simulink model "BTB_Case_v1"  (R2021a)
settings: Solver=FixedStepDiscrete  StartTime=0.0  StopTime=24  FixedStep=Ts_Power  RelTol=1e-3
InitFcn:
  | %Simulation parameters
  | Ts_Power = 50e-6;
  | Ts_Control = 50e-6;
  | Ts_sec = 0.05;
  | 
  | %MV Grid parameters
  | U1n = 20e3;
  | f = 50;
  | omega = 2*pi*50;
  | 
  | 
  | %LCL filter parameters
  | L_t = 100e-6;
  | C = 173e-6;
  | L_s = 100e-6;
  | R_d = 0.086;
  | R_t = omega*L_t/100;
  | R_s = omega*L_s/100;
  | 
  | %Capacitance of the DC bus
  | Cdc = 5.88e-3;
  | Rdc = 0.00001;
  | 
  | %Coupling transformers parameters
  | U2n = 400;
  | Sn1 = 3e6;
  | 
  | %Primary Subestation parameters
  | Un = 110e3;
  | Sn = 30e6;
  | 
  | %Feeder parameters
  | Le_line_1 = 12; %length km
  | R_line_1 = (0.337)*Le_line_1; %Resistance ohms
  | X_line_1 = (0.358)*Le_line_1; %Reactance ohms
  | L_line_1 = X_line_1/omega;%Inductance H
  | 
  | Le_line_2 = 10; %length km
  | R_line_2 = (0.337)*Le_line_2; %Resistance ohms
  | X_line_2 = (0.358)*Le_line_2; %Reactance ohms
  | L_line_2 = X_line_2/omega; %Inductance H
  | 
  | %PLL parameters
  | K_p_pll = 1.8;
  | K_i_pll = 1.8/0.00251;
  | 
  | %Current control loop gains
  | tau_c = 3e-3;
  | L = L_t + L_s;
  | R =R_t + R_s;
  | Kp = L/tau_c;
  | Ki = R/tau_c;
  | 
  | %DC bus voltage control loop gains
  | tau_dc = 3*tau_c;
  | 
  | %Q-V primary control loop
  | RQ = 0.15; %Q-V regulation constant
  | 
  | %24-hours household profile pu
  | t_profile = [0:1:24].';
  | p_profile_h = [0.26 0.2 0.19 0.19 0.19 0.25 0.4 0.6 0.64 0.64 0.67 0.6 0.73 0.63 0.57 0.5 0.47 0.65 0.8 0.93 0.82 0.67 0.55 0.38 0.26].';
  | fdp_h = 0.87;
  | fi_h = acos(fdp_h);
  | q_profile_h = p_profile_h*tan(fi_h);
  | S_h = 3e6;
  | 
  | %24-hours industrial profile pu
  | p_profile_i = [0.33 0.32 0.29 0.32 0.37 0.45 0.67 0.88 1 0.99 1 0.79 0.83 0.83 0.83 0.8 0.55 0.65 0.5 0.46 0.41 0.4 0.36 0.36 0.33].';
  | fdp_i = 0.98;
  | fi_i = acos(fdp_h);
  | q_profile_i = p_profile_i*tan(fi_i);
  | S_i = 3e6;
  | 
  | %24-hours PV profile pu
  | p_profile_pv = [0 0 0 0 0 0 0 0 0 0.03 0.12 0.14 0.15 0.12 0.11 0.10 0.09 0.07 0.04 0 0 0 0 0 0].'*1/0.15;
  | S_pv = 6e6;
  | 
  | %24-hours WT profile pu
  | p_profile_wt = [0.9 0.9 1.1 1 0.9 1.1 1.25 1 0.9 0.8 0.9 0.9 1 0.8 1.5 1.3 1.2 1.2 1 0.7 1.2 0.9 1.3 1.4 0.9].'*1/1.5;
  | S_wt= 8e6;
undefined symbols (not defined in the file): D11, Delta, DiscIntNeverNeededParam, V
libraries: spsThreePhaseSeriesRLCBranchLib x16, spsThreePhaseVIMeasurementLib x13, spsRMSLib x10, simulink x6, spsSeriesRLCBranchLib x4, spsThreePhaseTransformerTwoWindingsLib x4, spsThreePhaseDynamicLoadLib x4, spsPower3phInstantaneousLib x3, eeGeneralControl x2, spsUniversalBridgeLib x2, spsVoltageMeasurementLib x2, spsThreePhaseSourceLib x1
(part 1 of 2)
settings Model: Creator=Manuel  LastModifiedBy=Manuel_Barragan

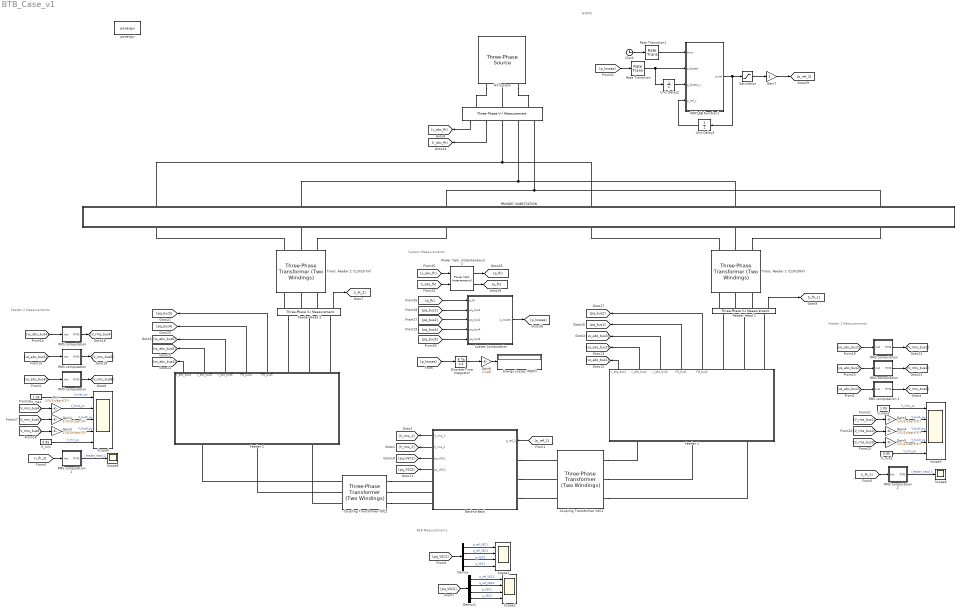
== system BTB_Case_v1 ==
  note: Feeder 2 Measurements
  note: Feeder 1 Measurements
  note: System Measurements
  note: A-DMS
  note: B2B Measurements
  " " : spsThreePhaseVIMeasurementLib/Three-Phase V-I Measurement  VoltageMeasurement=phase-to-ground  SetLabelV=off  LabelV=Vabc  Vpu=off  VpuLL=off  CurrentMeasurement=yes  SetLabelI=off  LabelI=Iabc  Ipu=off  Pbase=100e6  Vbase=500e3  OutputType=Complex  PhasorSimulation=off  PSBequivalent=0
  Back-to-Back : Subsystem
  Clock : Clock
  "Coupling Transformer VSC1 " : spsThreePhaseTransformerTwoWindingsLib/Three-Phase Transformer (Two Windings)  Winding1Connection=Delta (D11)  Winding2Connection=Yg  CoreType=Three single-phase transformers  SetSaturation=off  Hysteresis=off  DataFile='hysteresis'  SetInitialFlux=off  Measurements=None  UNITS=pu  NominalPower=[ Sn1 , f ]  Winding1=[ U1n , 0.002 , 0.08 ]  Winding2=[ U2n , 0.002 , 0.08 ]  Rm=500  Lm=500  L0=0.5  Saturation=[ 0,0 ; 0.0024,1.2 ; 1.0,1.52 ]  InitialFluxes=[ 0.8 , -0.8 , 0.7 ]  BreakLoop=off  DiscreteSolver=Trapezoidal iterative  DataType=off  TransfoNumber=1
  Coupling Transformer VSC2 : spsThreePhaseTransformerTwoWindingsLib/Three-Phase Transformer (Two Windings)  Winding1Connection=Delta (D11)  Winding2Connection=Yg  CoreType=Three single-phase transformers  SetSaturation=off  Hysteresis=off  DataFile='hysteresis'  SetInitialFlux=off  Measurements=None  UNITS=pu  NominalPower=[ Sn1 , f ]  Winding1=[ U1n , 0.002 , 0.08 ]  Winding2=[ U2n , 0.002 , 0.08 ]  Rm=500  Lm=500  L0=0.5  Saturation=[ 0,0 ; 0.0024,1.2 ; 1.0,1.52 ]  InitialFluxes=[ 0.8 , -0.8 , 0.7 ]  BreakLoop=off  DiscreteSolver=Trapezoidal iterative  DataType=off  TransfoNumber=1
  Demux : Demux
  Demux1 : Demux
  Discrete-Time Integrator : DiscreteIntegrator  SampleTime=Ts_Control  ICPrevOutput=DiscIntNeverNeededParam  ICPrevScaledInput=DiscIntNeverNeededParam
  Energy Losses (MWh) : Display
  Feeder 1 : Subsystem
  Feeder 2 : Subsystem
  Feeder Head 1 : spsThreePhaseVIMeasurementLib/Three-Phase V-I Measurement  VoltageMeasurement=no  SetLabelV=off  LabelV=Vabc  Vpu=off  VpuLL=off  CurrentMeasurement=yes  SetLabelI=off  LabelI=Iabc  Ipu=off  Pbase=100e6  Vbase=500e3  OutputType=Complex  PhasorSimulation=off  PSBequivalent=0
  Feeder Head 2 : spsThreePhaseVIMeasurementLib/Three-Phase V-I Measurement  VoltageMeasurement=no  SetLabelV=off  LabelV=Vabc  Vpu=off  VpuLL=off  CurrentMeasurement=yes  SetLabelI=off  LabelI=Iabc  Ipu=off  Pbase=100e6  Vbase=500e3  OutputType=Complex  PhasorSimulation=off  PSBequivalent=0
  Gain{,1..5} (6 alike) : Gain  Gain=1/(U1n/sqrt(3))
  Gain6 : Gain  Gain=1/1e6
  Gain7 : Gain
  HV System : spsThreePhaseSourceLib/Three-Phase Source  InternalConnection=Yg  VoltagePhases=off  Voltage=Un  PhaseAngle=0  Voltage_phases=[25e3 25e3 25e3]/sqrt(3)  PhaseAngles_phases=[0 -120 +120]  Frequency=f  NonIdealSource=off  SpecifyImpedance=on  Resistance=0.8929  Inductance=16.58e-3  ShortCircuitLevel=100e6  BaseVoltage=V  XRratio=7  BusType=swing  Pref=10e3  Qref=0  Prefabc=[10e3, 10e3, 10e3]  Qrefabc=[0, 0, 0]  Qmin=-inf  Qmax=inf
  Losses Computation : MATLAB Function  TreatAsAtomicUnit=on
  MATLAB Function1 : MATLAB Function  TreatAsAtomicUnit=on
  PRIMARY SUBESTATION : Subsystem
  "Power (3ph, Instantaneous)1" : spsPower3phInstantaneousLib/Power (3ph, Instantaneous)
  RMS computation : Subsystem
  "RMS computation " : Subsystem
  "RMS computation  " : Subsystem
  "RMS computation   " : Subsystem
  "RMS computation    " : Subsystem
  RMS computation  1 : Subsystem
  RMS computation  2 : Subsystem
  RMS computation 1 : Subsystem
  Rate Transition : RateTransition  InitialCondition=Ts_sec
  Rate Transition1 : RateTransition  InitialCondition=Ts_sec
  Saturation : Saturate  UpperLimit=Sn1  LowerLimit=-Sn1
  Scope1 : Scope  NumInputPorts=4
  Scope2 : Scope  NumInputPorts=4
  Scope3 : Scope  NumInputPorts=5
  Scope4 : Scope  NumInputPorts=5
  Scope5 : Scope
  Scope6 : Scope
  Trans. Feeder 1 (110/20kV) : spsThreePhaseTransformerTwoWindingsLib/Three-Phase Transformer (Two Windings)  Winding1Connection=Yg  Winding2Connection=Yg  CoreType=Three single-phase transformers  SetSaturation=off  Hysteresis=off  DataFile='hysteresis'  SetInitialFlux=off  Measurements=None  UNITS=pu  NominalPower=[ Sn , f ]  Winding1=[ Un , 0.002 , 0.08 ]  Winding2=[ U1n , 0.002 , 0.08 ]  Rm=500  Lm=500  L0=0.5  Saturation=[ 0,0 ; 0.0024,1.2 ; 1.0,1.52 ]  InitialFluxes=[ 0.8 , -0.8 , 0.7 ]  BreakLoop=off  DiscreteSolver=Trapezoidal iterative  DataType=off  TransfoNumber=1
  Trans. Feeder 2 (110/20 kV) : spsThreePhaseTransformerTwoWindingsLib/Three-Phase Transformer (Two Windings)  Winding1Connection=Yg  Winding2Connection=Yg  CoreType=Three single-phase transformers  SetSaturation=off  Hysteresis=off  DataFile='hysteresis'  SetInitialFlux=off  Measurements=None  UNITS=pu  NominalPower=[Sn , f ]  Winding1=[ Un , 0.002 , 0.08 ]  Winding2=[ U1n , 0.002 , 0.08 ]  Rm=500  Lm=500  L0=0.5  Saturation=[ 0,0 ; 0.0024,1.2 ; 1.0,1.52 ]  InitialFluxes=[ 0.8 , -0.8 , 0.7 ]  BreakLoop=off  DiscreteSolver=Trapezoidal iterative  DataType=off  TransfoNumber=1
  Unit Delay2 : UnitDelay  SampleTime=Ts_sec  HasFrameUpgradeWarning=on
  Unit Delay3 : UnitDelay  SampleTime=Ts_sec  HasFrameUpgradeWarning=on
  V_max : Constant  Value=1.05
  V_max2 : Constant  Value=1.05
  V_min : Constant  Value=0.95
  V_min2 : Constant  Value=0.95
  powergui : spspowerguiLib/powergui  Priority=1  SimulationMode=Discrete  SampleTime=Ts_Power  frequency=60  Iterations=50  frequencyindice=50  Pbase=100e6  ErrMax=1e-4  UnitsV=kV  UnitsW=MW  buscounter=0  FunctionMessages=off  echomessages=off  EnableUseOfTLC=off  CurrentSourceSwitches=off  DisableSnubberDevices=off  DisableRonSwitches=off  DisableVfSwitches=off  DisplayEquations=off  AutomaticDiscreteSolvers=off  SolverType=Tustin/Backward Euler (TBE)  Interpol=off  ExternalGateDelay=off  methode=off  Ts=100  x0status=blocks  SPID=on  SwTol=0  HookPort=off  NonlinearTolerance=1e-4  nMaxIteration=100  ContinueOnMaxIteration=off  RestoreLinks=warning  ResistiveCurrentMeasurement=off  Frange=[0:2:500]  Ylog=off  Xlog=on  ShowGrid=off  save=off  variable=ZData  structure=0  ZoomFFT=off  StartTime=0.0  cycles=1  DisplayStyle=1  fundamental=60  FreqAxis=off  MaxFrequency=1000  frequencyindicesteady=1  RmsSteady=1  display=off
  wires:
  Feeder 1/1(v_abc_bus1) -> [vs_abc_bus1]
  Feeder 1/2(v_abc_bus2) -> [vs_abc_bus2]
  Feeder 1/4(PQ_bus1) -> [pq_bus1]
  Feeder 1/5(PQ_bus2) -> [pq_bus2]
  Feeder 2/1(v_abc_bus4) -> [vs_abc_bus4]
  Feeder 2/2(v_abc_bus5) -> [vs_abc_bus5]
  Feeder 2/4(PQ_bus4) -> [pq_bus4]
  Feeder 2/5(PQ_bus5) -> [pq_bus5]
  [vs_abc_bus4] -> "RMS computation  "/1(Inst)
  "RMS computation  "/1(RMS) -> [V_rms_bus4]
  "RMS computation   "/1(RMS) -> [V_rms_bus5]
  [vs_abc_bus5] -> "RMS computation   "/1(Inst)
  [vs_abc_bus2] -> "RMS computation "/1(Inst)
  "RMS computation "/1(RMS) -> [V_rms_bus2]
  RMS computation/1(RMS) -> [V_rms_bus1]
  [vs_abc_bus1] -> RMS computation/1(Inst)
  [V_rms_bus4] -> Gain/1
  Gain/1 -> Scope4/2  "V_bus4_pu"
  Gain1/1 -> Scope4/3  "V_bus5_pu"
  [V_rms_bus5] -> Gain1/1
  Gain2/1 -> Scope4/4  "V_bus6_pu"
  [V_rms_bus6] -> Gain2/1
  [V_rms_bus3] -> Gain5/1
  Gain5/1 -> Scope3/4  "V_bus3_pu"
  [V_rms_bus2] -> Gain4/1
  Gain4/1 -> Scope3/3  "V_bus2_pu"
  Gain3/1 -> Scope3/2  "V_bus1_pu"
  [V_rms_bus1] -> Gain3/1
  [i_abc_fh] -> "Power (3ph, Instantaneous)1"/2
  [v_abc_fh] -> "Power (3ph, Instantaneous)1"/1
  "Power (3ph, Instantaneous)1"/1 -> [p_fh]
  "Power (3ph, Instantaneous)1"/2 -> [q_fh]
  " "/1 -> [v_abc_fh]
  " "/2 -> [i_abc_fh]
  Unit Delay2/1 -> MATLAB Function1/3(p_losses_z)
  MATLAB Function1/1(p_ref) -> Saturation/1, Unit Delay3/1
  Unit Delay3/1 -> MATLAB Function1/4(p_ref_z)
  Clock/1 -> Rate Transition1/1
  [p_losses] -> Rate Transition/1
  Rate Transition/1 -> Unit Delay2/1, MATLAB Function1/2(p_losses)
  Rate Transition1/1 -> MATLAB Function1/1(time)
  Saturation/1 -> Gain7/1
  Back-to-Back/2(V_rms_2) -> [V_rms_2]
  Back-to-Back/1(V_rms_1) -> [V_rms_1]
  [p_ref_2] -> Back-to-Back/1(p_ref_2)
  [p_fh] -> Losses Computation/1(p_fh)
  Losses Computation/1(p_losses) -> [p_losses]
  [pq_bus1] -> Losses Computation/2(pq_bus1)
  [pq_bus2] -> Losses Computation/3(pq_bus2)
  [p_losses] -> Discrete-Time Integrator/1
  Discrete-Time Integrator/1 -> Gain6/1
  Gain6/1 -> Energy Losses (MWh)/1
  Gain7/1 -> [p_ref_2]
  Feeder 1/3(v_abc_bus3) -> [vs_abc_bus3]
  RMS computation 1/1(RMS) -> [V_rms_bus3]
  [vs_abc_bus3] -> RMS computation 1/1(Inst)
  Feeder 2/3(v_abc_bus6) -> [vs_abc_bus6]
  [pq_bus4] -> Losses Computation/4(pq_bus4)
  [pq_bus5] -> Losses Computation/5(pq_bus5)
  [vs_abc_bus6] -> "RMS computation    "/1(Inst)
  "RMS computation    "/1(RMS) -> [V_rms_bus6]
  V_max/1 -> Scope4/1  "V_max_pu"
  V_min/1 -> Scope4/5  "V_min_pu"
  V_max2/1 -> Scope3/1  "V_max_pu"
  V_min2/1 -> Scope3/5  "V_min_pu"
  Feeder Head 2/1 -> [i_fh_2]
  Feeder Head 1/1 -> [i_fh_1]
  [i_fh_2] -> RMS computation  1/1(Inst)
  RMS computation  1/1(RMS) -> Scope5/1  "I_feeder_head_2"
  RMS computation  2/1(RMS) -> Scope6/1  "I_feeder_head_1"
  [i_fh_1] -> RMS computation  2/1(Inst)
  Back-to-Back/3(pq_VSC1) -> [pq_VSC1]
  Back-to-Back/4(pq_VSC2) -> [pq_VSC2]
  [pq_VSC1] -> Demux/1
  Demux/1 -> Scope1/1  "p_ref_VSC1"
  Demux/2 -> Scope1/2  "q_ref_VSC1"
  Demux/3 -> Scope1/3  "p_VSC1"
  Demux/4 -> Scope1/4  "q_VSC1"
  Demux1/1 -> Scope2/1  "p_ref_VSC2"
  Demux1/2 -> Scope2/2  "q_ref_VSC2"
  [pq_VSC2] -> Demux1/1
  Demux1/4 -> Scope2/4  "q_VSC2"
  Demux1/3 -> Scope2/3  "p_VSC2"
  connections:
  "Coupling Transformer VSC1 "/LConn1 -- Feeder 1/LConn1
  "Coupling Transformer VSC1 "/LConn2 -- Feeder 1/LConn2
  "Coupling Transformer VSC1 "/LConn3 -- Feeder 1/LConn3
  Trans. Feeder 2 (110/20 kV)/LConn1 -- PRIMARY SUBESTATION/RConn1
  Trans. Feeder 2 (110/20 kV)/LConn2 -- PRIMARY SUBESTATION/RConn2
  Trans. Feeder 2 (110/20 kV)/LConn3 -- PRIMARY SUBESTATION/RConn3
  Trans. Feeder 1 (110/20kV)/LConn1 -- PRIMARY SUBESTATION/RConn4
  Trans. Feeder 1 (110/20kV)/LConn2 -- PRIMARY SUBESTATION/RConn5
  Trans. Feeder 1 (110/20kV)/LConn3 -- PRIMARY SUBESTATION/RConn6
  Coupling Transformer VSC2/LConn1 -- Feeder 2/LConn1
  Coupling Transformer VSC2/LConn2 -- Feeder 2/LConn2
  Coupling Transformer VSC2/LConn3 -- Feeder 2/LConn3
  " "/LConn2 -- HV System/RConn2
  HV System/RConn1 -- " "/LConn1
  HV System/RConn3 -- " "/LConn3
  Coupling Transformer VSC2/RConn1 -- Back-to-Back/RConn1
  Back-to-Back/LConn1 -- "Coupling Transformer VSC1 "/RConn1
  Coupling Transformer VSC2/RConn2 -- Back-to-Back/RConn2
  Back-to-Back/LConn2 -- "Coupling Transformer VSC1 "/RConn2
  Coupling Transformer VSC2/RConn3 -- Back-to-Back/RConn3
  Back-to-Back/LConn3 -- "Coupling Transformer VSC1 "/RConn3
  Feeder Head 2/RConn2 -- Trans. Feeder 2 (110/20 kV)/RConn2
  Feeder Head 2/RConn1 -- Trans. Feeder 2 (110/20 kV)/RConn3
  Feeder Head 2/LConn1 -- Feeder 2/RConn3
  Feeder Head 2/LConn2 -- Feeder 2/RConn2
  Feeder Head 2/LConn3 -- Feeder 2/RConn1
  Feeder Head 2/RConn3 -- Trans. Feeder 2 (110/20 kV)/RConn1
  Feeder Head 1/RConn2 -- Trans. Feeder 1 (110/20kV)/RConn2
  Feeder Head 1/RConn1 -- Trans. Feeder 1 (110/20kV)/RConn3
  Feeder Head 1/RConn3 -- Trans. Feeder 1 (110/20kV)/RConn1
  Feeder Head 1/LConn3 -- Feeder 1/RConn1
  Feeder Head 1/LConn2 -- Feeder 1/RConn2
  Feeder Head 1/LConn1 -- Feeder 1/RConn3
  " "/RConn1 -- PRIMARY SUBESTATION/LConn4 -- PRIMARY SUBESTATION/LConn1
  PRIMARY SUBESTATION/LConn2 -- PRIMARY SUBESTATION/LConn5 -- " "/RConn2
  PRIMARY SUBESTATION/LConn3 -- PRIMARY SUBESTATION/LConn6 -- " "/RConn3

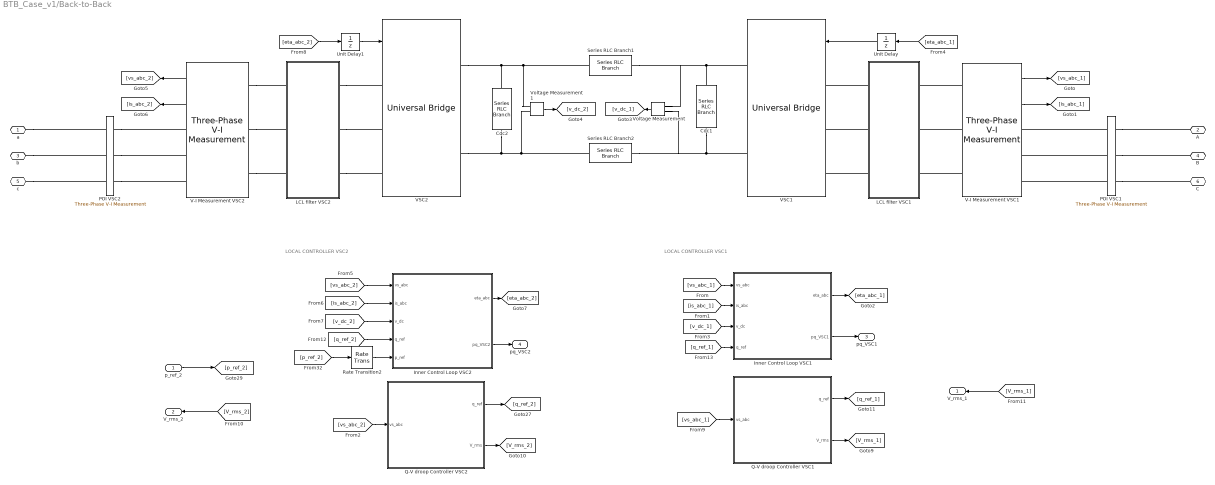
== system BTB_Case_v1/Back-to-Back ==
  note: LOCAL CONTROLLER VSC2
  note: LOCAL CONTROLLER VSC1
  p_ref_2 : Inport
  Cdc1 : spsSeriesRLCBranchLib/Series RLC Branch  LConnTagsString=__new0  RConnTagsString=__new0  BranchType=C  Resistance=1  Inductance=1e-3  SetiL0=off  InitialCurrent=0  Capacitance=Cdc  Setx0=on  InitialVoltage=U2n*sqrt(2)  Measurements=None
  Cdc2 : spsSeriesRLCBranchLib/Series RLC Branch  LConnTagsString=__new0  RConnTagsString=__new0  BranchType=C  Resistance=1  Inductance=1e-3  SetiL0=off  InitialCurrent=0  Capacitance=Cdc  Setx0=on  InitialVoltage=U2n*sqrt(2)  Measurements=None
  Inner Control Loop VSC1 : Subsystem
  Inner Control Loop VSC2 : Subsystem
  LCL filter VSC1 : Subsystem
  LCL filter VSC2 : Subsystem
  POI VSC1 : spsThreePhaseVIMeasurementLib/Three-Phase V-I Measurement  VoltageMeasurement=no  SetLabelV=off  LabelV=Vabc  Vpu=off  VpuLL=off  CurrentMeasurement=no  SetLabelI=off  LabelI=Iabc  Ipu=off  Pbase=100e6  Vbase=500e3  OutputType=Complex  PhasorSimulation=off  PSBequivalent=0
  POI VSC2 : spsThreePhaseVIMeasurementLib/Three-Phase V-I Measurement  VoltageMeasurement=no  SetLabelV=off  LabelV=Vabc  Vpu=off  VpuLL=off  CurrentMeasurement=no  SetLabelI=off  LabelI=Iabc  Ipu=off  Pbase=100e6  Vbase=500e3  OutputType=Complex  PhasorSimulation=off  PSBequivalent=0
  Q-V droop Controller VSC1 : Subsystem
  Q-V droop Controller VSC2 : Subsystem
  Rate Transition2 : RateTransition  InitialCondition=Ts_Control
  Series RLC Branch1 : spsSeriesRLCBranchLib/Series RLC Branch  LConnTagsString=__new0  RConnTagsString=__new0  BranchType=R  Resistance=Rdc  Inductance=1e-3  SetiL0=off  InitialCurrent=0  Capacitance=C  Setx0=on  InitialVoltage=V*sqrt(2)  Measurements=None
  Series RLC Branch2 : spsSeriesRLCBranchLib/Series RLC Branch  LConnTagsString=__new0  RConnTagsString=__new0  BranchType=R  Resistance=Rdc  Inductance=1e-3  SetiL0=off  InitialCurrent=0  Capacitance=C  Setx0=on  InitialVoltage=V*sqrt(2)  Measurements=None
  Unit Delay : UnitDelay  SampleTime=Ts_Power  HasFrameUpgradeWarning=on
  Unit Delay1 : UnitDelay  SampleTime=Ts_Power  HasFrameUpgradeWarning=on
  V-I Measurement VSC1 : spsThreePhaseVIMeasurementLib/Three-Phase V-I Measurement  VoltageMeasurement=phase-to-ground  SetLabelV=off  LabelV=Vabc  Vpu=off  VpuLL=off  CurrentMeasurement=yes  SetLabelI=off  LabelI=Iabc  Ipu=off  Pbase=100e6  Vbase=500e3  OutputType=Complex  PhasorSimulation=off  PSBequivalent=0
  V-I Measurement VSC2 : spsThreePhaseVIMeasurementLib/Three-Phase V-I Measurement  VoltageMeasurement=phase-to-ground  SetLabelV=off  LabelV=Vabc  Vpu=off  VpuLL=off  CurrentMeasurement=yes  SetLabelI=off  LabelI=Iabc  Ipu=off  Pbase=100e6  Vbase=500e3  OutputType=Complex  PhasorSimulation=off  PSBequivalent=0
  VSC1 : spsUniversalBridgeLib/Universal Bridge  Arms=3  SnubberResistance=1e5  SnubberCapacitance=inf  Device=Average-model based VSC  Ron=1e-3  Lon=0  ForwardVoltages="[  0  0  ]"  ForwardVoltage=0  GTOparameters=[ 10e-6 , 20e-6 ]  IGBTparameters=[ 1e-6 , 2e-6 ]  Measurements=None  Measurements_2=None  converterType=Rectifier
  VSC2 : spsUniversalBridgeLib/Universal Bridge  Arms=3  SnubberResistance=1e5  SnubberCapacitance=inf  Device=Average-model based VSC  Ron=1e-3  Lon=0  ForwardVoltages="[  0  0  ]"  ForwardVoltage=0  GTOparameters=[ 10e-6 , 20e-6 ]  IGBTparameters=[ 1e-6 , 2e-6 ]  Measurements=None  Measurements_2=None  converterType=Rectifier
  Voltage Measurement : spsVoltageMeasurementLib/Voltage Measurement  PhasorSimulation=off  OutputType=Complex  PSBequivalent=0
  Voltage Measurement1 : spsVoltageMeasurementLib/Voltage Measurement  PhasorSimulation=off  OutputType=Complex  PSBequivalent=0
  a : PMIOPort  Side=Right
  A : PMIOPort  Port=2  Side=Left
  b : PMIOPort  Port=3  Side=Right
  B : PMIOPort  Port=4  Side=Left
  c : PMIOPort  Port=5  Side=Right
  C : PMIOPort  Port=6  Side=Left
  V_rms_1 : Outport
  V_rms_2 : Outport  Port=2
  pq_VSC1 : Outport  Port=3
  pq_VSC2 : Outport  Port=4
  wires:
  Voltage Measurement1/1 -> [v_dc_2]
  [eta_abc_1] -> Unit Delay/1
  V-I Measurement VSC1/2 -> [is_abc_1]
  V-I Measurement VSC2/2 -> [is_abc_2]
  Unit Delay/1 -> VSC1/1
  V-I Measurement VSC2/1 -> [vs_abc_2]
  [eta_abc_2] -> Unit Delay1/1
  V-I Measurement VSC1/1 -> [vs_abc_1]
  Unit Delay1/1 -> VSC2/1
  Voltage Measurement/1 -> [v_dc_1]
  Q-V droop Controller VSC2/2(V_rms) -> [V_rms_2]
  Rate Transition2/1 -> Inner Control Loop VSC2/5(p_ref)
  [q_ref_2] -> Inner Control Loop VSC2/4(q_ref)
  [p_ref_2] -> Rate Transition2/1
  Inner Control Loop VSC2/1(eta_abc) -> [eta_abc_2]
  Q-V droop Controller VSC2/1(q_ref) -> [q_ref_2]
  [v_dc_2] -> Inner Control Loop VSC2/3(v_dc)
  [vs_abc_2] -> Inner Control Loop VSC2/1(vs_abc)
  [vs_abc_2] -> Q-V droop Controller VSC2/1(vs_abc)
  [is_abc_2] -> Inner Control Loop VSC2/2(is_abc)
  [v_dc_1] -> Inner Control Loop VSC1/3(v_dc)
  Q-V droop Controller VSC1/1(q_ref) -> [q_ref_1]
  [V_rms_1] -> V_rms_1/1
  [vs_abc_1] -> Q-V droop Controller VSC1/1(vs_abc)
  [q_ref_1] -> Inner Control Loop VSC1/4(q_ref)
  Q-V droop Controller VSC1/2(V_rms) -> [V_rms_1]
  [is_abc_1] -> Inner Control Loop VSC1/2(is_abc)
  Inner Control Loop VSC1/1(eta_abc) -> [eta_abc_1]
  [vs_abc_1] -> Inner Control Loop VSC1/1(vs_abc)
  [V_rms_2] -> V_rms_2/1
  p_ref_2/1 -> [p_ref_2]
  Inner Control Loop VSC1/2(pq_VSC1) -> pq_VSC1/1
  Inner Control Loop VSC2/2(pq_VSC2) -> pq_VSC2/1
  connections:
  Cdc1/LConn1 -- VSC1/RConn1 -- Series RLC Branch1/LConn1 -- Voltage Measurement/LConn1
  LCL filter VSC1/LConn3 -- VSC1/LConn3
  POI VSC1/RConn1 -- V-I Measurement VSC1/RConn1
  c/RConn1 -- POI VSC2/RConn3
  V-I Measurement VSC2/LConn1 -- LCL filter VSC2/RConn1
  LCL filter VSC2/LConn2 -- VSC2/LConn2
  Cdc1/RConn1 -- VSC1/RConn2 -- Voltage Measurement/LConn2 -- Series RLC Branch2/LConn1
  V-I Measurement VSC1/LConn3 -- LCL filter VSC1/RConn3
  V-I Measurement VSC1/LConn2 -- LCL filter VSC1/RConn2
  V-I Measurement VSC1/LConn1 -- LCL filter VSC1/RConn1
  LCL filter VSC2/LConn1 -- VSC2/LConn1
  Cdc2/RConn1 -- Voltage Measurement1/LConn2 -- Series RLC Branch2/RConn1 -- VSC2/RConn2
  POI VSC2/LConn2 -- V-I Measurement VSC2/RConn2
  Cdc2/LConn1 -- Voltage Measurement1/LConn1 -- Series RLC Branch1/RConn1 -- VSC2/RConn1
  POI VSC2/LConn1 -- V-I Measurement VSC2/RConn1
  POI VSC2/LConn3 -- V-I Measurement VSC2/RConn3
  LCL filter VSC1/LConn1 -- VSC1/LConn1
  V-I Measurement VSC2/LConn3 -- LCL filter VSC2/RConn3
  LCL filter VSC1/LConn2 -- VSC1/LConn2
  LCL filter VSC2/LConn3 -- VSC2/LConn3
  POI VSC1/RConn2 -- V-I Measurement VSC1/RConn2
  POI VSC1/LConn1 -- A/RConn1
  POI VSC1/RConn3 -- V-I Measurement VSC1/RConn3
  V-I Measurement VSC2/LConn2 -- LCL filter VSC2/RConn2
  b/RConn1 -- POI VSC2/RConn2
  a/RConn1 -- POI VSC2/RConn1
  POI VSC1/LConn2 -- B/RConn1
  POI VSC1/LConn3 -- C/RConn1

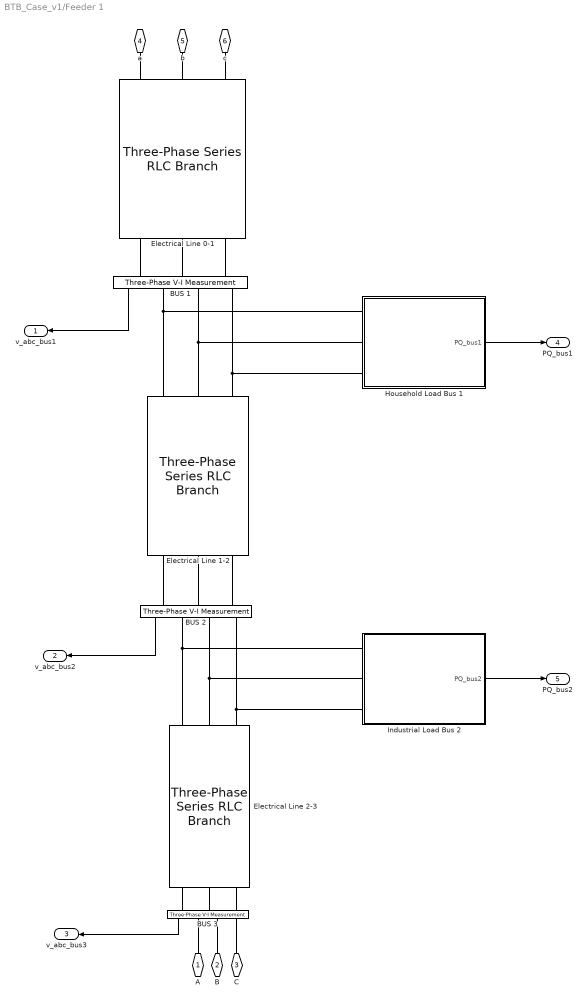
== system BTB_Case_v1/Feeder 1 ==
  BUS 1 : spsThreePhaseVIMeasurementLib/Three-Phase V-I Measurement  VoltageMeasurement=phase-to-ground  SetLabelV=off  LabelV=Vabc  Vpu=off  VpuLL=off  CurrentMeasurement=no  SetLabelI=off  LabelI=Iabc  Ipu=off  Pbase=100e6  Vbase=500e3  OutputType=Complex  PhasorSimulation=off  PSBequivalent=0
  BUS 2 : spsThreePhaseVIMeasurementLib/Three-Phase V-I Measurement  VoltageMeasurement=phase-to-ground  SetLabelV=off  LabelV=Vabc  Vpu=off  VpuLL=off  CurrentMeasurement=no  SetLabelI=off  LabelI=Iabc  Ipu=off  Pbase=100e6  Vbase=500e3  OutputType=Complex  PhasorSimulation=off  PSBequivalent=0
  BUS 3 : spsThreePhaseVIMeasurementLib/Three-Phase V-I Measurement  VoltageMeasurement=phase-to-ground  SetLabelV=off  LabelV=Vabc  Vpu=off  VpuLL=off  CurrentMeasurement=no  SetLabelI=off  LabelI=Iabc  Ipu=off  Pbase=100e6  Vbase=500e3  OutputType=Complex  PhasorSimulation=off  PSBequivalent=0
  Electrical Line 0-1 : spsThreePhaseSeriesRLCBranchLib/Three-Phase Series RLC Branch  LConnTagsString=A|B|C  RConnTagsString=A|B|C  BranchType=RL  Resistance=R_line_1*0.35  Inductance=L_line_1*0.35  Capacitance=1e-6  Measurements=None
  Electrical Line 1-2 : spsThreePhaseSeriesRLCBranchLib/Three-Phase Series RLC Branch  LConnTagsString=A|B|C  RConnTagsString=A|B|C  BranchType=RL  Resistance=R_line_1/2  Inductance=L_line_1/2  Capacitance=1e-6  Measurements=None
  Electrical Line 2-3 : spsThreePhaseSeriesRLCBranchLib/Three-Phase Series RLC Branch  LConnTagsString=A|B|C  RConnTagsString=A|B|C  BranchType=RL  Resistance=R_line_1*0.15  Inductance=L_line_1*0.15  Capacitance=1e-6  Measurements=None
  Household Load Bus 1 : Subsystem
  Industrial Load Bus 2 : Subsystem
  A : PMIOPort  Side=Left
  B : PMIOPort  Port=2  Side=Left
  C : PMIOPort  Port=3  Side=Left
  a : PMIOPort  Port=4  Side=Right
  b : PMIOPort  Port=5  Side=Right
  c : PMIOPort  Port=6  Side=Right
  v_abc_bus1 : Outport
  v_abc_bus2 : Outport  Port=2
  v_abc_bus3 : Outport  Port=3
  PQ_bus1 : Outport  Port=4
  PQ_bus2 : Outport  Port=5
  wires:
  BUS 1/1 -> v_abc_bus1/1
  BUS 2/1 -> v_abc_bus2/1
  Household Load Bus 1/1(PQ_bus1) -> PQ_bus1/1
  Industrial Load Bus 2/1(PQ_bus2) -> PQ_bus2/1
  BUS 3/1 -> v_abc_bus3/1
  connections:
  b/RConn1 -- Electrical Line 0-1/RConn2
  BUS 1/LConn3 -- Electrical Line 0-1/LConn3
  a/RConn1 -- Electrical Line 0-1/RConn1
  c/RConn1 -- Electrical Line 0-1/RConn3
  BUS 1/LConn2 -- Electrical Line 0-1/LConn2
  BUS 1/LConn1 -- Electrical Line 0-1/LConn1
  BUS 2/LConn1 -- Electrical Line 1-2/LConn1
  BUS 2/LConn2 -- Electrical Line 1-2/LConn2
  BUS 2/LConn3 -- Electrical Line 1-2/LConn3
  Electrical Line 1-2/RConn1 -- Household Load Bus 1/LConn1 -- BUS 1/RConn1
  Electrical Line 1-2/RConn2 -- Household Load Bus 1/LConn2 -- BUS 1/RConn2
  Electrical Line 1-2/RConn3 -- Household Load Bus 1/LConn3 -- BUS 1/RConn3
  Electrical Line 2-3/RConn2 -- Industrial Load Bus 2/LConn2 -- BUS 2/RConn2
  Electrical Line 2-3/RConn1 -- Industrial Load Bus 2/LConn1 -- BUS 2/RConn1
  Electrical Line 2-3/RConn3 -- BUS 2/RConn3 -- Industrial Load Bus 2/LConn3
  BUS 3/LConn2 -- Electrical Line 2-3/LConn2
  BUS 3/LConn1 -- Electrical Line 2-3/LConn1
  BUS 3/LConn3 -- Electrical Line 2-3/LConn3
  C/RConn1 -- BUS 3/RConn3
  B/RConn1 -- BUS 3/RConn2
  A/RConn1 -- BUS 3/RConn1

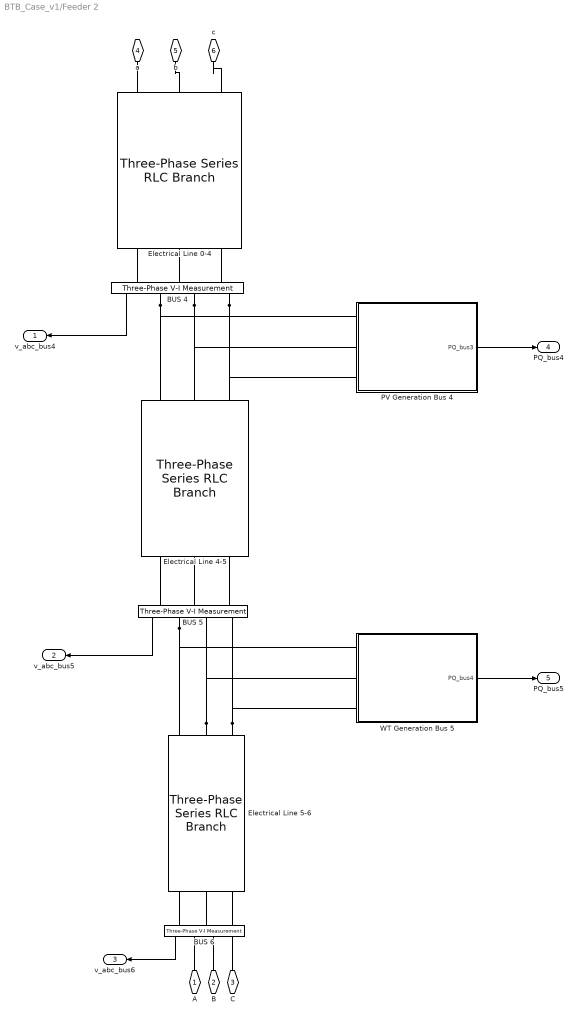
== system BTB_Case_v1/Feeder 2 ==
  BUS 4 : spsThreePhaseVIMeasurementLib/Three-Phase V-I Measurement  VoltageMeasurement=phase-to-ground  SetLabelV=off  LabelV=Vabc  Vpu=off  VpuLL=off  CurrentMeasurement=no  SetLabelI=off  LabelI=Iabc  Ipu=off  Pbase=100e6  Vbase=500e3  OutputType=Complex  PhasorSimulation=off  PSBequivalent=0
  BUS 5 : spsThreePhaseVIMeasurementLib/Three-Phase V-I Measurement  VoltageMeasurement=phase-to-ground  SetLabelV=off  LabelV=Vabc  Vpu=off  VpuLL=off  CurrentMeasurement=no  SetLabelI=off  LabelI=Iabc  Ipu=off  Pbase=100e6  Vbase=500e3  OutputType=Complex  PhasorSimulation=off  PSBequivalent=0
  BUS 6 : spsThreePhaseVIMeasurementLib/Three-Phase V-I Measurement  VoltageMeasurement=phase-to-ground  SetLabelV=off  LabelV=Vabc  Vpu=off  VpuLL=off  CurrentMeasurement=no  SetLabelI=off  LabelI=Iabc  Ipu=off  Pbase=100e6  Vbase=500e3  OutputType=Complex  PhasorSimulation=off  PSBequivalent=0
  Electrical Line 0-4 : spsThreePhaseSeriesRLCBranchLib/Three-Phase Series RLC Branch  LConnTagsString=A|B|C  RConnTagsString=A|B|C  BranchType=RL  Resistance=R_line_2*0.3  Inductance=L_line_2*0.3  Capacitance=1e-6  Measurements=None
  Electrical Line 4-5 : spsThreePhaseSeriesRLCBranchLib/Three-Phase Series RLC Branch  LConnTagsString=A|B|C  RConnTagsString=A|B|C  BranchType=RL  Resistance=R_line_2*0.5  Inductance=L_line_2*0.5  Capacitance=1e-6  Measurements=None
  Electrical Line 5-6 : spsThreePhaseSeriesRLCBranchLib/Three-Phase Series RLC Branch  LConnTagsString=A|B|C  RConnTagsString=A|B|C  BranchType=RL  Resistance=R_line_2*0.2  Inductance=L_line_2*0.2  Capacitance=1e-6  Measurements=None
  PV Generation Bus 4 : Subsystem
  WT Generation Bus 5 : Subsystem
  A : PMIOPort  Side=Left
  B : PMIOPort  Port=2  Side=Left
  C : PMIOPort  Port=3  Side=Left
  a : PMIOPort  Port=4  Side=Right
  b : PMIOPort  Port=5  Side=Right
  c : PMIOPort  Port=6  Side=Right
  v_abc_bus4 : Outport
  v_abc_bus5 : Outport  Port=2
  v_abc_bus6 : Outport  Port=3
  PQ_bus4 : Outport  Port=4
  PQ_bus5 : Outport  Port=5
  wires:
  WT Generation Bus 5/1(PQ_bus4) -> PQ_bus5/1
  PV Generation Bus 4/1(PQ_bus3) -> PQ_bus4/1
  BUS 5/1 -> v_abc_bus5/1
  BUS 4/1 -> v_abc_bus4/1
  BUS 6/1 -> v_abc_bus6/1
  connections:
  BUS 5/LConn3 -- Electrical Line 4-5/LConn3
  BUS 5/LConn2 -- Electrical Line 4-5/LConn2
  BUS 5/LConn1 -- Electrical Line 4-5/LConn1
  BUS 4/RConn3 -- Electrical Line 4-5/RConn3 -- PV Generation Bus 4/LConn3
  BUS 4/RConn2 -- Electrical Line 4-5/RConn2 -- PV Generation Bus 4/LConn2
  BUS 4/RConn1 -- Electrical Line 4-5/RConn1 -- PV Generation Bus 4/LConn1
  BUS 4/LConn1 -- Electrical Line 0-4/LConn1
  BUS 4/LConn2 -- Electrical Line 0-4/LConn2
  c/RConn1 -- Electrical Line 0-4/RConn3
  a/RConn1 -- Electrical Line 0-4/RConn1
  BUS 4/LConn3 -- Electrical Line 0-4/LConn3
  b/RConn1 -- Electrical Line 0-4/RConn2
  BUS 5/RConn1 -- WT Generation Bus 5/LConn1 -- Electrical Line 5-6/RConn1
  Electrical Line 5-6/RConn3 -- BUS 5/RConn3 -- WT Generation Bus 5/LConn3
  Electrical Line 5-6/RConn2 -- BUS 5/RConn2 -- WT Generation Bus 5/LConn2
  BUS 6/LConn2 -- Electrical Line 5-6/LConn2
  BUS 6/LConn3 -- Electrical Line 5-6/LConn3
  BUS 6/LConn1 -- Electrical Line 5-6/LConn1
  BUS 6/RConn3 -- C/RConn1
  B/RConn1 -- BUS 6/RConn2
  A/RConn1 -- BUS 6/RConn1

== system BTB_Case_v1/PRIMARY SUBESTATION ==
  a1 : PMIOPort  Side=Right
  b1 : PMIOPort  Port=2  Side=Right
  c1 : PMIOPort  Port=3  Side=Right
  A1 : PMIOPort  Port=4  Side=Left
  B1 : PMIOPort  Port=5  Side=Left
  C1 : PMIOPort  Port=6  Side=Left
  A2 : PMIOPort  Port=7  Side=Left
  B2 : PMIOPort  Port=8  Side=Left
  C2 : PMIOPort  Port=9  Side=Left
  a2 : PMIOPort  Port=10  Side=Right
  b2 : PMIOPort  Port=11  Side=Right
  c2 : PMIOPort  Port=12  Side=Right
  connections:
  a1/RConn1 -- A1/RConn1
  b1/RConn1 -- B1/RConn1
  c1/RConn1 -- C1/RConn1
  a2/RConn1 -- A2/RConn1
  b2/RConn1 -- B2/RConn1
  c2/RConn1 -- C2/RConn1

== system BTB_Case_v1/RMS computation ==
  Inst : Inport
  Demux1 : Demux  Outputs=3
  RMS1 : spsRMSLib/RMS  TrueRMS=on  Freq=f  RMSInit=U2n/sqrt(3)  Ts=Ts_Control
  RMS : Outport
  wires:
  RMS1/1 -> RMS/1
  Inst/1 -> Demux1/1
  Demux1/1 -> RMS1/1

== system BTB_Case_v1/RMS computation  ==
  Inst : Inport
  Demux1 : Demux  Outputs=3
  RMS1 : spsRMSLib/RMS  TrueRMS=on  Freq=f  RMSInit=U2n/sqrt(3)  Ts=Ts_Control
  RMS : Outport
  wires:
  RMS1/1 -> RMS/1
  Inst/1 -> Demux1/1
  Demux1/1 -> RMS1/1

== system BTB_Case_v1/RMS computation   ==
  Inst : Inport
  Demux1 : Demux  Outputs=3
  RMS1 : spsRMSLib/RMS  TrueRMS=on  Freq=f  RMSInit=U2n/sqrt(3)  Ts=Ts_Control
  RMS : Outport
  wires:
  RMS1/1 -> RMS/1
  Inst/1 -> Demux1/1
  Demux1/1 -> RMS1/1

== system BTB_Case_v1/RMS computation    ==
  Inst : Inport
  Demux1 : Demux  Outputs=3
  RMS1 : spsRMSLib/RMS  TrueRMS=on  Freq=f  RMSInit=U2n/sqrt(3)  Ts=Ts_Control
  RMS : Outport
  wires:
  RMS1/1 -> RMS/1
  Inst/1 -> Demux1/1
  Demux1/1 -> RMS1/1

== system BTB_Case_v1/RMS computation     ==
  Inst : Inport
  Demux1 : Demux  Outputs=3
  RMS1 : spsRMSLib/RMS  TrueRMS=on  Freq=f  RMSInit=U2n/sqrt(3)  Ts=Ts_Control
  RMS : Outport
  wires:
  Demux1/1 -> RMS1/1
  Inst/1 -> Demux1/1
  RMS1/1 -> RMS/1

== system BTB_Case_v1/RMS computation  1 ==
  Inst : Inport
  Demux1 : Demux  Outputs=3
  RMS1 : spsRMSLib/RMS  TrueRMS=on  Freq=f  RMSInit=U2n/sqrt(3)  Ts=Ts_Control
  RMS : Outport
  wires:
  Demux1/1 -> RMS1/1
  Inst/1 -> Demux1/1
  RMS1/1 -> RMS/1

== system BTB_Case_v1/RMS computation  2 ==
  Inst : Inport
  Demux1 : Demux  Outputs=3
  RMS1 : spsRMSLib/RMS  TrueRMS=on  Freq=f  RMSInit=U2n/sqrt(3)  Ts=Ts_Control
  RMS : Outport
  wires:
  Demux1/1 -> RMS1/1
  Inst/1 -> Demux1/1
  RMS1/1 -> RMS/1

== system BTB_Case_v1/RMS computation 1 ==
  Inst : Inport
  Demux1 : Demux  Outputs=3
  RMS1 : spsRMSLib/RMS  TrueRMS=on  Freq=f  RMSInit=U2n/sqrt(3)  Ts=Ts_Control
  RMS : Outport
  wires:
  RMS1/1 -> RMS/1
  Inst/1 -> Demux1/1
  Demux1/1 -> RMS1/1

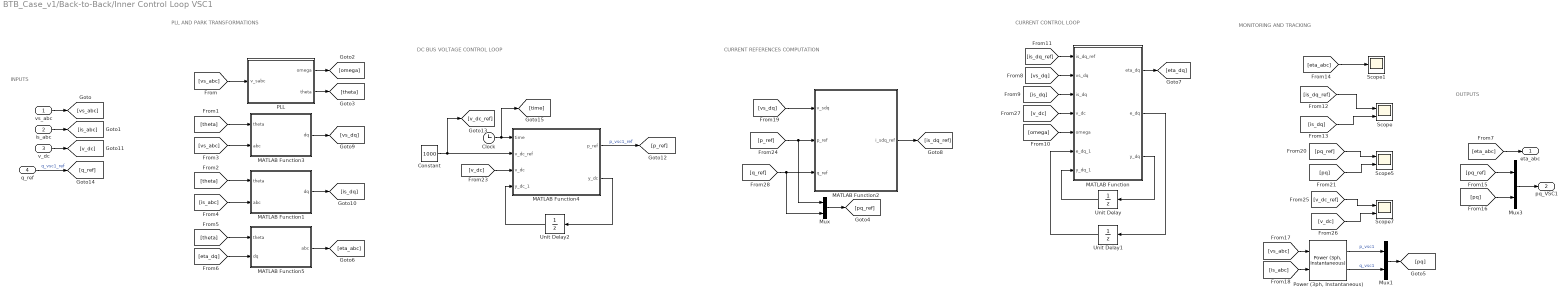
== system BTB_Case_v1/Back-to-Back/Inner Control Loop VSC1 ==
  note: INPUTS
  note: PLL AND PARK TRANSFORMATIONS
  note: DC BUS VOLTAGE CONTROL LOOP
  note: CURRENT REFERENCES COMPUTATION
  note: MONITORING AND TRACKING
  note: OUTPUTS
  note: CURRENT CONTROL LOOP
  vs_abc : Inport
  is_abc : Inport  Port=2
  v_dc : Inport  Port=3
  q_ref : Inport  Port=4
  Clock : Clock
  Constant : Constant  Value=1000
  MATLAB Function : MATLAB Function  TreatAsAtomicUnit=on
  MATLAB Function1 : MATLAB Function  TreatAsAtomicUnit=on
  MATLAB Function2 : MATLAB Function  TreatAsAtomicUnit=on
  MATLAB Function3 : MATLAB Function  TreatAsAtomicUnit=on
  MATLAB Function4 : MATLAB Function  TreatAsAtomicUnit=on
  MATLAB Function5 : MATLAB Function  TreatAsAtomicUnit=on
  Mux : Mux  Inputs=2
  Mux1 : Mux  Inputs=2
  Mux3 : Mux  Inputs=2
  PLL : Subsystem
  "Power (3ph, Instantaneous)" : spsPower3phInstantaneousLib/Power (3ph, Instantaneous)
  Scope : Scope  NumInputPorts=2
  Scope1 : Scope
  Scope5 : Scope  NumInputPorts=2
  Scope7 : Scope  NumInputPorts=2
  Unit Delay : UnitDelay  InitialCondition=[0;0]  SampleTime=Ts_Control  HasFrameUpgradeWarning=on
  Unit Delay1 : UnitDelay  InitialCondition=[0;0]  SampleTime=Ts_Control  HasFrameUpgradeWarning=on
  Unit Delay2 : UnitDelay  SampleTime=Ts_Control  HasFrameUpgradeWarning=on
  eta_abc : Outport
  pq_VSC1 : Outport  Port=2
  wires:
  vs_abc/1 -> [vs_abc]
  is_abc/1 -> [is_abc]
  [vs_abc] -> PLL/1(v_sabc)
  PLL/1(omega) -> [omega]
  PLL/2(theta) -> [theta]
  [theta] -> MATLAB Function3/1(theta)
  [theta] -> MATLAB Function1/1(theta)
  [vs_abc] -> MATLAB Function3/2(abc)
  [is_abc] -> MATLAB Function1/2(abc)
  MATLAB Function3/1(dq) -> [vs_dq]
  MATLAB Function1/1(dq) -> [is_dq]
  [theta] -> MATLAB Function5/1(theta)
  [eta_dq] -> MATLAB Function5/2(dq)
  MATLAB Function5/1(abc) -> [eta_abc]
  [eta_abc] -> eta_abc/1
  [is_dq_ref] -> Scope/1
  [is_dq] -> Scope/2
  [eta_abc] -> Scope1/1
  [vs_abc] -> "Power (3ph, Instantaneous)"/1
  [is_abc] -> "Power (3ph, Instantaneous)"/2
  "Power (3ph, Instantaneous)"/1 -> Mux1/1  "p_vsc1"
  "Power (3ph, Instantaneous)"/2 -> Mux1/2  "q_vsc1"
  MATLAB Function2/1(i_sdq_ref) -> [is_dq_ref]
  [vs_dq] -> MATLAB Function2/1(v_sdq)
  [p_ref] -> Mux/1, MATLAB Function2/2(p_ref)
  [q_ref] -> Mux/2, MATLAB Function2/3(q_ref)
  Mux/1 -> [pq_ref]
  Mux1/1 -> [pq]
  [pq_ref] -> Scope5/1
  [pq] -> Scope5/2
  MATLAB Function4/2(y_dc) -> Unit Delay2/1
  Unit Delay2/1 -> MATLAB Function4/4(y_dc_1)
  v_dc/1 -> [v_dc]
  [v_dc] -> MATLAB Function4/3(v_dc)
  Constant/1 -> [v_dc_ref], MATLAB Function4/2(v_dc_ref)
  MATLAB Function4/1(p_ref) -> [p_ref]  "p_vsc1_ref"
  [v_dc_ref] -> Scope7/1
  [v_dc] -> Scope7/2
  Clock/1 -> [time], MATLAB Function4/1(time)
  [is_dq_ref] -> MATLAB Function/1(is_dq_ref)
  [omega] -> MATLAB Function/5(omega)
  Unit Delay1/1 -> MATLAB Function/6(e_dq_1)
  MATLAB Function/1(eta_dq) -> [eta_dq]
  Unit Delay/1 -> MATLAB Function/7(y_dq_1)
  [vs_dq] -> MATLAB Function/2(vs_dq)
  MATLAB Function/3(y_dq) -> Unit Delay/1
  [is_dq] -> MATLAB Function/3(is_dq)
  MATLAB Function/2(e_dq) -> Unit Delay1/1
  [v_dc] -> MATLAB Function/4(v_dc)
  q_ref/1 -> [q_ref]  "q_vsc1_ref"
  [pq] -> Mux3/2
  Mux3/1 -> pq_VSC1/1
  [pq_ref] -> Mux3/1

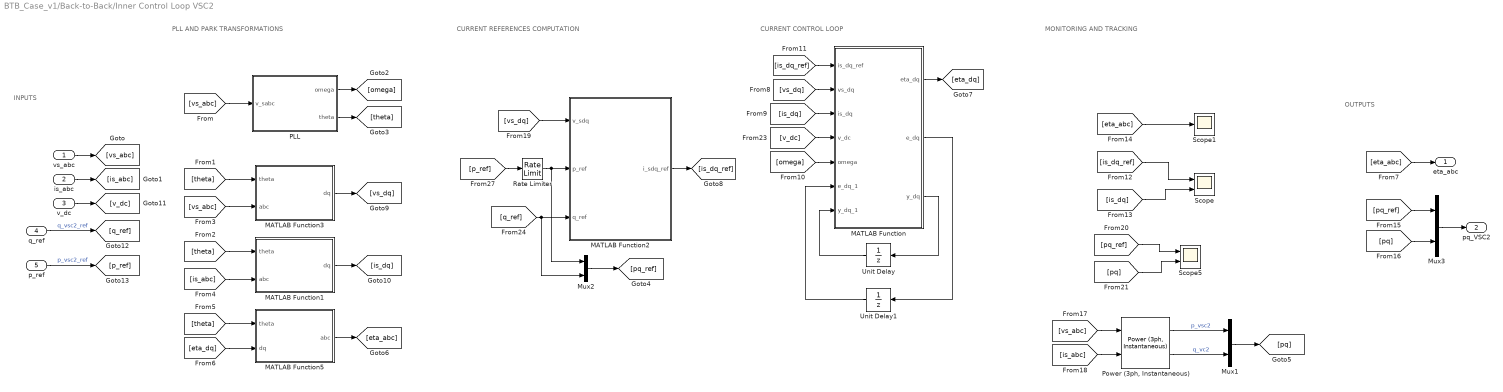
== system BTB_Case_v1/Back-to-Back/Inner Control Loop VSC2 ==
  note: MONITORING AND TRACKING
  note: CURRENT CONTROL LOOP
  note: CURRENT REFERENCES COMPUTATION
  note: INPUTS
  note: PLL AND PARK TRANSFORMATIONS
  note: OUTPUTS
  vs_abc : Inport
  is_abc : Inport  Port=2
  v_dc : Inport  Port=3
  q_ref : Inport  Port=4
  p_ref : Inport  Port=5
  MATLAB Function : MATLAB Function  TreatAsAtomicUnit=on
  MATLAB Function1 : MATLAB Function  TreatAsAtomicUnit=on
  MATLAB Function2 : MATLAB Function  TreatAsAtomicUnit=on
  MATLAB Function3 : MATLAB Function  TreatAsAtomicUnit=on
  MATLAB Function5 : MATLAB Function  TreatAsAtomicUnit=on
  Mux1 : Mux  Inputs=2
  Mux2 : Mux  Inputs=2
  Mux3 : Mux  Inputs=2
  PLL : Subsystem
  "Power (3ph, Instantaneous)" : spsPower3phInstantaneousLib/Power (3ph, Instantaneous)
  Rate Limiter : RateLimiter  RisingSlewLimit=500e3  FallingSlewLimit=-500e3  SampleTimeMode=inherited
  Scope : Scope  NumInputPorts=2
  Scope1 : Scope
  Scope5 : Scope  NumInputPorts=2
  Unit Delay : UnitDelay  InitialCondition=[0;0]  SampleTime=Ts_Control  HasFrameUpgradeWarning=on
  Unit Delay1 : UnitDelay  InitialCondition=[0;0]  SampleTime=Ts_Control  HasFrameUpgradeWarning=on
  eta_abc : Outport
  pq_VSC2 : Outport  Port=2
  wires:
  v_dc/1 -> [v_dc]
  [pq] -> Scope5/2
  [pq_ref] -> Scope5/1
  Mux1/1 -> [pq]
  [q_ref] -> Mux2/2, MATLAB Function2/3(q_ref)
  [vs_dq] -> MATLAB Function2/1(v_sdq)
  MATLAB Function2/1(i_sdq_ref) -> [is_dq_ref]
  Unit Delay1/1 -> MATLAB Function/6(e_dq_1)
  MATLAB Function/2(e_dq) -> Unit Delay1/1
  Unit Delay/1 -> MATLAB Function/7(y_dq_1)
  MATLAB Function/3(y_dq) -> Unit Delay/1
  "Power (3ph, Instantaneous)"/2 -> Mux1/2  "q_vc2"
  "Power (3ph, Instantaneous)"/1 -> Mux1/1  "p_vsc2"
  [is_abc] -> "Power (3ph, Instantaneous)"/2
  [vs_abc] -> "Power (3ph, Instantaneous)"/1
  [eta_abc] -> Scope1/1
  [is_dq] -> Scope/2
  [is_dq_ref] -> Scope/1
  [is_dq_ref] -> MATLAB Function/1(is_dq_ref)
  MATLAB Function/1(eta_dq) -> [eta_dq]
  [omega] -> MATLAB Function/5(omega)
  [is_dq] -> MATLAB Function/3(is_dq)
  [vs_dq] -> MATLAB Function/2(vs_dq)
  [eta_abc] -> eta_abc/1
  MATLAB Function5/1(abc) -> [eta_abc]
  [eta_dq] -> MATLAB Function5/2(dq)
  [theta] -> MATLAB Function5/1(theta)
  MATLAB Function1/1(dq) -> [is_dq]
  MATLAB Function3/1(dq) -> [vs_dq]
  [is_abc] -> MATLAB Function1/2(abc)
  [vs_abc] -> MATLAB Function3/2(abc)
  [theta] -> MATLAB Function1/1(theta)
  [theta] -> MATLAB Function3/1(theta)
  PLL/2(theta) -> [theta]
  PLL/1(omega) -> [omega]
  [vs_abc] -> PLL/1(v_sabc)
  is_abc/1 -> [is_abc]
  vs_abc/1 -> [vs_abc]
  [v_dc] -> MATLAB Function/4(v_dc)
  Mux2/1 -> [pq_ref]
  q_ref/1 -> [q_ref]  "q_vsc2_ref"
  p_ref/1 -> [p_ref]  "p_vsc2_ref"
  [p_ref] -> Rate Limiter/1
  Rate Limiter/1 -> Mux2/1, MATLAB Function2/2(p_ref)
  Mux3/1 -> pq_VSC2/1
  [pq_ref] -> Mux3/1
  [pq] -> Mux3/2

== system BTB_Case_v1/Back-to-Back/LCL filter VSC1 ==
  Three-Phase Series RLC Branch : spsThreePhaseSeriesRLCBranchLib/Three-Phase Series RLC Branch  LConnTagsString=A|B|C  RConnTagsString=A|B|C  BranchType=RL  Resistance=R_t  Inductance=L_t  Capacitance=1e-6  Measurements=None
  Three-Phase Series RLC Branch1 : spsThreePhaseSeriesRLCBranchLib/Three-Phase Series RLC Branch  LConnTagsString=A|B|C  RConnTagsString=A|B|C  BranchType=RL  Resistance=R_t  Inductance=L_t  Capacitance=1e-6  Measurements=None
  Three-Phase Series RLC Branch2 : spsThreePhaseSeriesRLCBranchLib/Three-Phase Series RLC Branch  LConnTagsString=A|B|C  RConnTagsString=A|B|C  BranchType=RC  Resistance=R_d  Inductance=L_t  Capacitance=C  Measurements=None
  A : PMIOPort  Side=Left
  B : PMIOPort  Port=2  Side=Left
  a : PMIOPort  Port=3  Side=Right
  C : PMIOPort  Port=4  Side=Left
  b : PMIOPort  Port=5  Side=Right
  c : PMIOPort  Port=6  Side=Right
  connections:
  Three-Phase Series RLC Branch/LConn3 -- C/RConn1
  Three-Phase Series RLC Branch/LConn2 -- B/RConn1
  Three-Phase Series RLC Branch/LConn1 -- A/RConn1
  Three-Phase Series RLC Branch1/LConn2 -- Three-Phase Series RLC Branch2/LConn2 -- Three-Phase Series RLC Branch/RConn2
  Three-Phase Series RLC Branch1/LConn3 -- Three-Phase Series RLC Branch2/LConn3 -- Three-Phase Series RLC Branch/RConn3
  Three-Phase Series RLC Branch1/LConn1 -- Three-Phase Series RLC Branch2/LConn1 -- Three-Phase Series RLC Branch/RConn1
  Three-Phase Series RLC Branch2/RConn1 -- Three-Phase Series RLC Branch2/RConn3 -- Three-Phase Series RLC Branch2/RConn2
  a/RConn1 -- Three-Phase Series RLC Branch1/RConn1
  b/RConn1 -- Three-Phase Series RLC Branch1/RConn2
  c/RConn1 -- Three-Phase Series RLC Branch1/RConn3

== system BTB_Case_v1/Back-to-Back/LCL filter VSC2 ==
  Three-Phase Series RLC Branch : spsThreePhaseSeriesRLCBranchLib/Three-Phase Series RLC Branch  LConnTagsString=A|B|C  RConnTagsString=A|B|C  BranchType=RL  Resistance=R_t  Inductance=L_t  Capacitance=1e-6  Measurements=None
  Three-Phase Series RLC Branch1 : spsThreePhaseSeriesRLCBranchLib/Three-Phase Series RLC Branch  LConnTagsString=A|B|C  RConnTagsString=A|B|C  BranchType=RL  Resistance=R_t  Inductance=L_t  Capacitance=1e-6  Measurements=None
  Three-Phase Series RLC Branch2 : spsThreePhaseSeriesRLCBranchLib/Three-Phase Series RLC Branch  LConnTagsString=A|B|C  RConnTagsString=A|B|C  BranchType=RC  Resistance=R_d  Inductance=L_t  Capacitance=C  Measurements=None
  A : PMIOPort  Side=Left
  B : PMIOPort  Port=2  Side=Left
  a : PMIOPort  Port=3  Side=Right
  C : PMIOPort  Port=4  Side=Left
  b : PMIOPort  Port=5  Side=Right
  c : PMIOPort  Port=6  Side=Right
  connections:
  c/RConn1 -- Three-Phase Series RLC Branch1/RConn3
  b/RConn1 -- Three-Phase Series RLC Branch1/RConn2
  a/RConn1 -- Three-Phase Series RLC Branch1/RConn1
  Three-Phase Series RLC Branch2/RConn3 -- Three-Phase Series RLC Branch2/RConn1 -- Three-Phase Series RLC Branch2/RConn2
  Three-Phase Series RLC Branch2/LConn1 -- Three-Phase Series RLC Branch1/LConn1 -- Three-Phase Series RLC Branch/RConn1
  Three-Phase Series RLC Branch2/LConn3 -- Three-Phase Series RLC Branch1/LConn3 -- Three-Phase Series RLC Branch/RConn3
  Three-Phase Series RLC Branch2/LConn2 -- Three-Phase Series RLC Branch1/LConn2 -- Three-Phase Series RLC Branch/RConn2
  Three-Phase Series RLC Branch/LConn1 -- A/RConn1
  Three-Phase Series RLC Branch/LConn2 -- B/RConn1
  Three-Phase Series RLC Branch/LConn3 -- C/RConn1

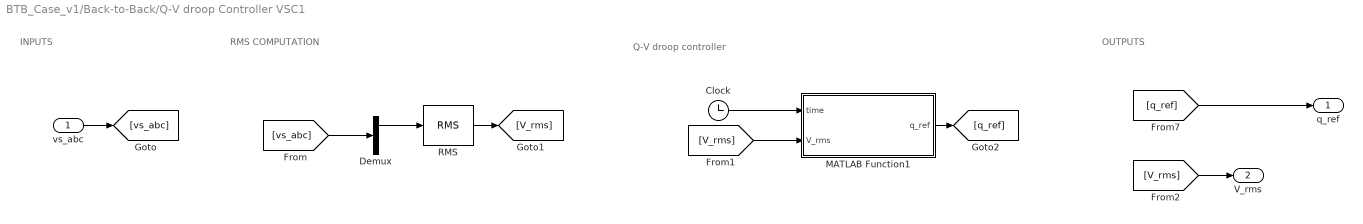
== system BTB_Case_v1/Back-to-Back/Q-V droop Controller VSC1 ==
  note: INPUTS
  note: RMS COMPUTATION
  note: OUTPUTS
  note: Q-V droop controller
  vs_abc : Inport
  Clock : Clock
  Demux : Demux  Outputs=3
  MATLAB Function1 : MATLAB Function  TreatAsAtomicUnit=on
  RMS : spsRMSLib/RMS  TrueRMS=on  Freq=f  RMSInit=U2n/sqrt(3)  Ts=Ts_Control
  q_ref : Outport
  V_rms : Outport  Port=2
  wires:
  vs_abc/1 -> [vs_abc]
  RMS/1 -> [V_rms]
  [vs_abc] -> Demux/1
  Demux/1 -> RMS/1
  [q_ref] -> q_ref/1
  [V_rms] -> V_rms/1
  Clock/1 -> MATLAB Function1/1(time)
  MATLAB Function1/1(q_ref) -> [q_ref]
  [V_rms] -> MATLAB Function1/2(V_rms)

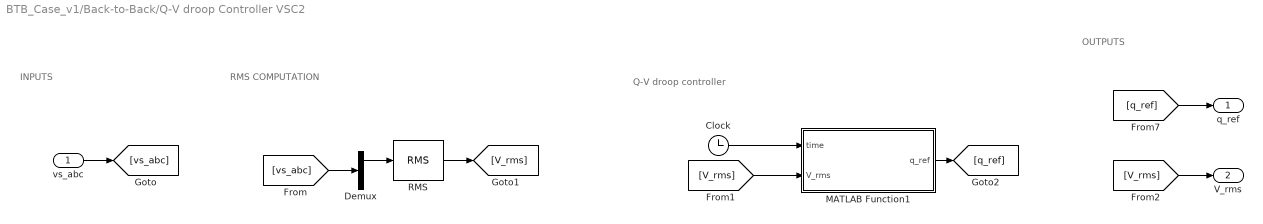
== system BTB_Case_v1/Back-to-Back/Q-V droop Controller VSC2 ==
  note: Q-V droop controller
  note: INPUTS
  note: RMS COMPUTATION
  note: OUTPUTS
  vs_abc : Inport
  Clock : Clock
  Demux : Demux  Outputs=3
  MATLAB Function1 : MATLAB Function  TreatAsAtomicUnit=on
  RMS : spsRMSLib/RMS  TrueRMS=on  Freq=f  RMSInit=U2n/sqrt(3)  Ts=Ts_Control
  q_ref : Outport
  V_rms : Outport  Port=2
  wires:
  vs_abc/1 -> [vs_abc]
  [vs_abc] -> Demux/1
  MATLAB Function1/1(q_ref) -> [q_ref]
  [V_rms] -> V_rms/1
  Demux/1 -> RMS/1
  RMS/1 -> [V_rms]
  [V_rms] -> MATLAB Function1/2(V_rms)
  [q_ref] -> q_ref/1
  Clock/1 -> MATLAB Function1/1(time)

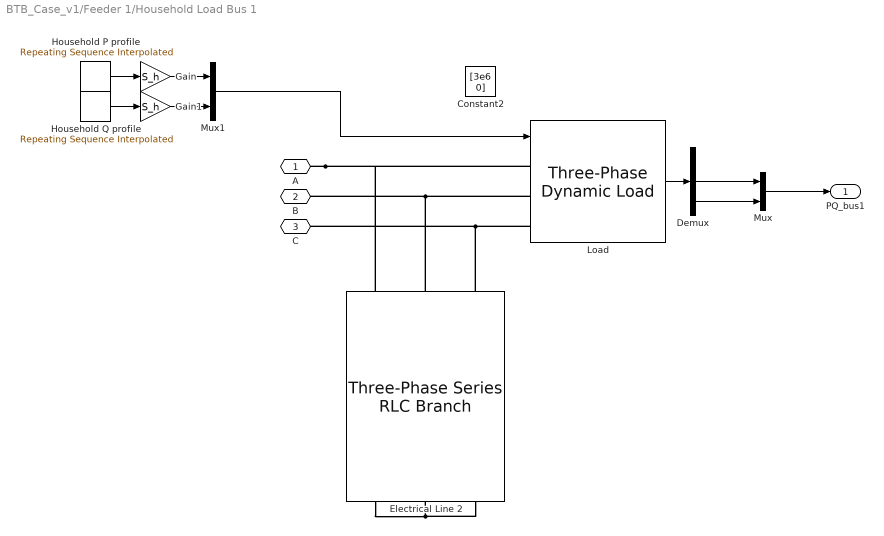
== system BTB_Case_v1/Feeder 1/Household Load Bus 1 ==
  Constant2 : Constant  Value=[3e6 0]
  Demux : Demux  Outputs=3
  Electrical Line 2 : spsThreePhaseSeriesRLCBranchLib/Three-Phase Series RLC Branch  LConnTagsString=A|B|C  RConnTagsString=A|B|C  BranchType=R  Resistance=1e6  Inductance=L_line_2/2  Capacitance=1e-6  Measurements=None
  Gain : Gain  Gain=S_h
  Gain1 : Gain  Gain=S_h
  Household P profile : simulink/Sources/Repeating Sequence Interpolated  OutValues=p_profile_h  TimeValues=t_profile  LookUpMeth=Interpolation-Use End Values  tsamp=Ts_Control  OutMin=[]  OutMax=[]  OutDataTypeStr=double  OutputDataTypeScalingMode=double  OutDataType=fixdt(0,8)  OutScaling=2^-10
  Household Q profile : simulink/Sources/Repeating Sequence Interpolated  OutValues=q_profile_h  TimeValues=t_profile  LookUpMeth=Interpolation-Use End Values  tsamp=Ts_Control  OutMin=[]  OutMax=[]  OutDataTypeStr=double  OutputDataTypeScalingMode=double  OutDataType=fixdt(0,8)  OutScaling=2^-10
  Load : spsThreePhaseDynamicLoadLib/Three-Phase Dynamic Load  NominalVoltage=[U1n f ]  ActiveReactivePowers=[0 0]  PositiveSequence=[1 0]  ExternalControl=on  NpNq=[1.3 2]  TimeConstants="[0  0  0  0]"  MinimumVoltage=0.7  Tfilter=1e-4  LoadFlowParameters=[4,0,0,0,0]
      settings: SourceProductBaseCode=PS
  Mux : Mux  Inputs=2
  Mux1 : Mux  Inputs=2
  A : PMIOPort  Side=Left
  B : PMIOPort  Port=2  Side=Left
  C : PMIOPort  Port=3  Side=Left
  PQ_bus1 : Outport
  wires:
  Load/1 -> Demux/1
  Demux/2 -> Mux/1
  Demux/3 -> Mux/2
  Mux/1 -> PQ_bus1/1
  Household P profile/1 -> Gain/1
  Gain/1 -> Mux1/1
  Gain1/1 -> Mux1/2
  Household Q profile/1 -> Gain1/1
  Mux1/1 -> Load/1
  connections:
  Electrical Line 2/LConn2 -- Load/LConn2 -- B/RConn1
  Electrical Line 2/LConn3 -- Load/LConn3 -- C/RConn1
  A/RConn1 -- Load/LConn1 -- Electrical Line 2/LConn1
  Electrical Line 2/RConn2 -- Electrical Line 2/RConn1 -- Electrical Line 2/RConn3

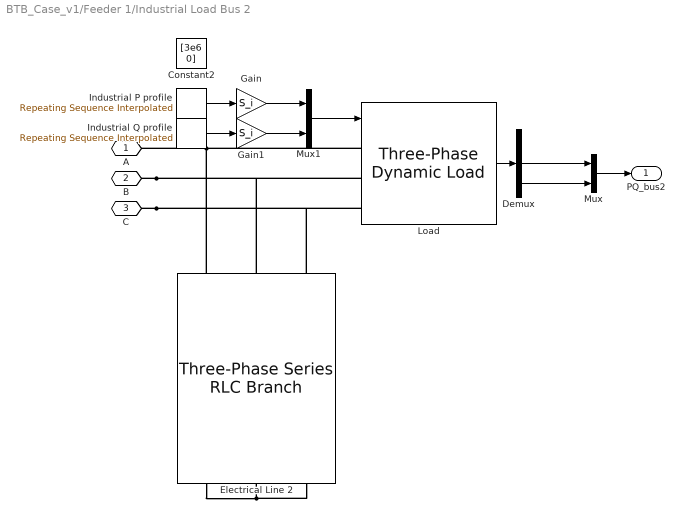
== system BTB_Case_v1/Feeder 1/Industrial Load Bus 2 ==
  Constant2 : Constant  Value=[3e6 0]
  Demux : Demux  Outputs=3
  Electrical Line 2 : spsThreePhaseSeriesRLCBranchLib/Three-Phase Series RLC Branch  LConnTagsString=A|B|C  RConnTagsString=A|B|C  BranchType=R  Resistance=1e6  Inductance=L_line_2/2  Capacitance=1e-6  Measurements=None
  Gain : Gain  Gain=S_i
  Gain1 : Gain  Gain=S_i
  Industrial P profile : simulink/Sources/Repeating Sequence Interpolated  OutValues=p_profile_i  TimeValues=t_profile  LookUpMeth=Interpolation-Use End Values  tsamp=Ts_Control  OutMin=[]  OutMax=[]  OutDataTypeStr=double  OutputDataTypeScalingMode=double  OutDataType=fixdt(0,8)  OutScaling=2^-10
  Industrial Q profile : simulink/Sources/Repeating Sequence Interpolated  OutValues=q_profile_i  TimeValues=t_profile  LookUpMeth=Interpolation-Use End Values  tsamp=Ts_Control  OutMin=[]  OutMax=[]  OutDataTypeStr=double  OutputDataTypeScalingMode=double  OutDataType=fixdt(0,8)  OutScaling=2^-10
  Load : spsThreePhaseDynamicLoadLib/Three-Phase Dynamic Load  NominalVoltage=[U1n f ]  ActiveReactivePowers=[0 0]  PositiveSequence=[1 0]  ExternalControl=on  NpNq=[1.3 2]  TimeConstants="[0  0  0  0]"  MinimumVoltage=0.7  Tfilter=1e-4  LoadFlowParameters=[4,0,0,0,0]
      settings: SourceProductBaseCode=PS
  Mux : Mux  Inputs=2
  Mux1 : Mux  Inputs=2
  A : PMIOPort  Side=Left
  B : PMIOPort  Port=2  Side=Left
  C : PMIOPort  Port=3  Side=Left
  PQ_bus2 : Outport
  wires:
  Load/1 -> Demux/1
  Mux/1 -> PQ_bus2/1
  Demux/3 -> Mux/2
  Demux/2 -> Mux/1
  Gain/1 -> Mux1/1
  Industrial P profile/1 -> Gain/1
  Gain1/1 -> Mux1/2
  Industrial Q profile/1 -> Gain1/1
  Mux1/1 -> Load/1
  connections:
  Electrical Line 2/RConn3 -- Electrical Line 2/RConn1 -- Electrical Line 2/RConn2
  Electrical Line 2/LConn1 -- Load/LConn1 -- A/RConn1
  C/RConn1 -- Load/LConn3 -- Electrical Line 2/LConn3
  B/RConn1 -- Load/LConn2 -- Electrical Line 2/LConn2

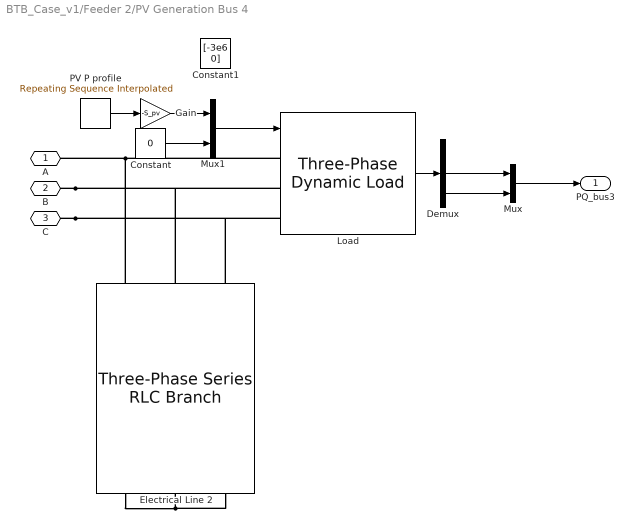
== system BTB_Case_v1/Feeder 2/PV Generation Bus 4 ==
  Constant : Constant  Value=0
  Constant1 : Constant  Value=[-3e6 0]
  Demux : Demux  Outputs=3
  Electrical Line 2 : spsThreePhaseSeriesRLCBranchLib/Three-Phase Series RLC Branch  LConnTagsString=A|B|C  RConnTagsString=A|B|C  BranchType=R  Resistance=1e6  Inductance=L_line_2/2  Capacitance=1e-6  Measurements=None
  Gain : Gain  Gain=-S_pv
  Load : spsThreePhaseDynamicLoadLib/Three-Phase Dynamic Load  NominalVoltage=[U1n f ]  ActiveReactivePowers=[0 0]  PositiveSequence=[1 0]  ExternalControl=on  NpNq=[1.3 2]  TimeConstants="[0  0  0  0]"  MinimumVoltage=0.7  Tfilter=1e-4  LoadFlowParameters=[4,0,0,0,0]
      settings: SourceProductBaseCode=PS
  Mux : Mux  Inputs=2
  Mux1 : Mux  Inputs=2
  PV P profile : simulink/Sources/Repeating Sequence Interpolated  OutValues=p_profile_pv  TimeValues=t_profile  LookUpMeth=Interpolation-Use End Values  tsamp=Ts_Control  OutMin=[]  OutMax=[]  OutDataTypeStr=double  OutputDataTypeScalingMode=double  OutDataType=fixdt(0,8)  OutScaling=2^-10
  A : PMIOPort  Side=Left
  B : PMIOPort  Port=2  Side=Left
  C : PMIOPort  Port=3  Side=Left
  PQ_bus3 : Outport
  wires:
  Mux/1 -> PQ_bus3/1
  Demux/3 -> Mux/2
  Demux/2 -> Mux/1
  Load/1 -> Demux/1
  PV P profile/1 -> Gain/1
  Gain/1 -> Mux1/1
  Constant/1 -> Mux1/2
  Mux1/1 -> Load/1
  connections:
  Electrical Line 2/RConn3 -- Electrical Line 2/RConn1 -- Electrical Line 2/RConn2
  Electrical Line 2/LConn1 -- Load/LConn1 -- A/RConn1
  C/RConn1 -- Load/LConn3 -- Electrical Line 2/LConn3
  B/RConn1 -- Load/LConn2 -- Electrical Line 2/LConn2

== system BTB_Case_v1/Feeder 2/WT Generation Bus 5 ==
  Constant : Constant  Value=0
  Constant1 : Constant  Value=[-3e6 0]
  Demux : Demux  Outputs=3
  Electrical Line 2 : spsThreePhaseSeriesRLCBranchLib/Three-Phase Series RLC Branch  LConnTagsString=A|B|C  RConnTagsString=A|B|C  BranchType=R  Resistance=1e6  Inductance=L_line_2/2  Capacitance=1e-6  Measurements=None
  Gain : Gain  Gain=-S_wt
  Load : spsThreePhaseDynamicLoadLib/Three-Phase Dynamic Load  NominalVoltage=[U1n f ]  ActiveReactivePowers=[0 0]  PositiveSequence=[1 0]  ExternalControl=on  NpNq=[1.3 2]  TimeConstants="[0  0  0  0]"  MinimumVoltage=0.7  Tfilter=1e-4  LoadFlowParameters=[4,0,0,0,0]
      settings: SourceProductBaseCode=PS
  Mux : Mux  Inputs=2
  Mux1 : Mux  Inputs=2
  WT P profile : simulink/Sources/Repeating Sequence Interpolated  OutValues=p_profile_wt  TimeValues=t_profile  LookUpMeth=Interpolation-Use End Values  tsamp=Ts_Control  OutMin=[]  OutMax=[]  OutDataTypeStr=double  OutputDataTypeScalingMode=double  OutDataType=fixdt(0,8)  OutScaling=2^-10
  A : PMIOPort  Side=Left
  B : PMIOPort  Port=2  Side=Left
  C : PMIOPort  Port=3  Side=Left
  PQ_bus4 : Outport
  wires:
  Demux/2 -> Mux/1
  Demux/3 -> Mux/2
  Mux/1 -> PQ_bus4/1
  Load/1 -> Demux/1
  WT P profile/1 -> Gain/1
  Gain/1 -> Mux1/1
  Constant/1 -> Mux1/2
  Mux1/1 -> Load/1
  connections:
  Electrical Line 2/LConn2 -- Load/LConn2 -- B/RConn1
  Electrical Line 2/LConn3 -- Load/LConn3 -- C/RConn1
  A/RConn1 -- Load/LConn1 -- Electrical Line 2/LConn1
  Electrical Line 2/RConn2 -- Electrical Line 2/RConn1 -- Electrical Line 2/RConn3

== system BTB_Case_v1/Back-to-Back/Inner Control Loop VSC1/PLL ==
  v_sabc : Inport
  Demux : Demux  Outputs=2
  Discrete-Time Integrator1 : DiscreteIntegrator  SampleTime=Ts_Control  ICPrevOutput=DiscIntNeverNeededParam  ICPrevScaledInput=DiscIntNeverNeededParam
  Integrator with Wrapped State (Discrete or Continuous) : eeGeneralControl/Integrator with Wrapped State (Discrete or Continuous)  LabelModeActiveChoice=Discrete  WrappedStateUpperValue=2*pi  WrappedStateLowerValue=0  x0=0  Ts=Ts_Control
      settings: SourceProductBaseCode=PS
  Ki : Gain  Gain=K_i_pll
  Kp : Gain  Gain=K_p_pll
  MATLAB Function1 : MATLAB Function  TreatAsAtomicUnit=on
  Sum : Sum  Inputs=|++
  omega : Outport  VectorParamsAs1DForOutWhenUnconnected=off
  theta : Outport  Port=2  VectorParamsAs1DForOutWhenUnconnected=off
  wires:
  MATLAB Function1/1(dq) -> [vs_dq], Demux/1
  v_sabc/1 -> MATLAB Function1/2(abc)
  Ki/1 -> Discrete-Time Integrator1/1
  Kp/1 -> Sum/1
  Discrete-Time Integrator1/1 -> Sum/2
  Sum/1 -> omega/1, Integrator with Wrapped State (Discrete or Continuous)/1
  Integrator with Wrapped State (Discrete or Continuous)/1 -> [theta], theta/1
  Demux/1 -> Ki/1, Kp/1  "v_sd"
  [theta] -> MATLAB Function1/1(theta)
